simulink model "untitled1"  (R2020a)
settings: Solver=VariableStepAuto  StartTime=0.0  StopTime=10  RelTol=1e-3
values from neighbouring files (symbols this model uses):
  A = [0 0 0 0 0 1 0 0 0 0 ... (first row only)    [Q3B.m]
  B = [0 0;0 0;0 0;0 0;0 0;0 0;0 0;0 0;0 0;Tem/m -1/m]    [Q3B.m]
  C = [0 0 0 0 1 0 0 0 0 0]    [Q3B.m]
  ca = 5*10^(-3)    (= 0.005)    [Q3B.m]
  D = [0 0]    [Q3B.m]
  J = 0.1*10^(-3)    (= 0.0001)    [Q3B.m]
  l = 280*10^(-6)    (= 0.00028)    [Q3B.m]
settings Model: Creator=Nir Lalum  LastModifiedBy=Nir Lalum
settings SFSimCC: CustomCodeUndefinedFunction=UseInterfaceOnly

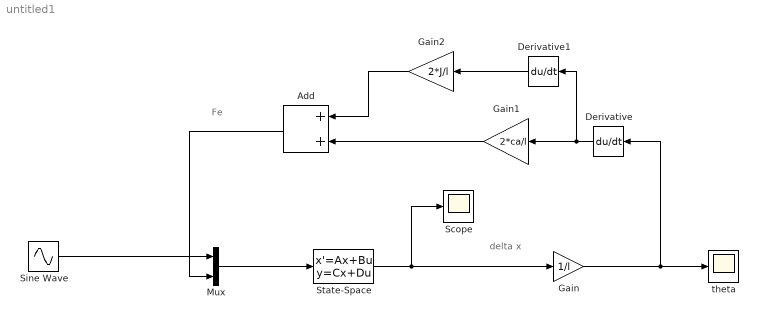
== system untitled1 ==
  note: Fe
  note: delta x
  Add : Sum
  Derivative : Derivative
  Derivative1 : Derivative
  Gain : Gain  Gain=1/l
  Gain1 : Gain  Gain=2*ca/l
  Gain2 : Gain  Gain=2*J/l
  Mux : Mux  Inputs=2
  Scope : Scope
  Sine Wave : Sin  Amplitude=50  Frequency=1200*pi  SampleTime=0
  State-Space : StateSpace  A=A  B=B  C=C  D=D  InitialCondition=1
  theta : Scope
  wires:
  Mux/1 -> State-Space/1
  State-Space/1 -> Gain/1, Scope/1
  Gain/1 -> Derivative/1, theta/1
  Derivative/1 -> Derivative1/1, Gain1/1
  Gain1/1 -> Add/2
  Derivative1/1 -> Gain2/1
  Gain2/1 -> Add/1
  Sine Wave/1 -> Mux/1
  Add/1 -> Mux/2
